simulink library "Custom_Valves"  (R2026a)
settings: Solver=VariableStepAuto
libraries: fl_lib x46, nesl_utility x7, MyMath_lib x2, SimscapeFluids_lib x2
Description:
  | Copyright 2020-2026 The MathWorks, Inc.
settings Model: Creator=smiller  LastModifiedBy=smiller

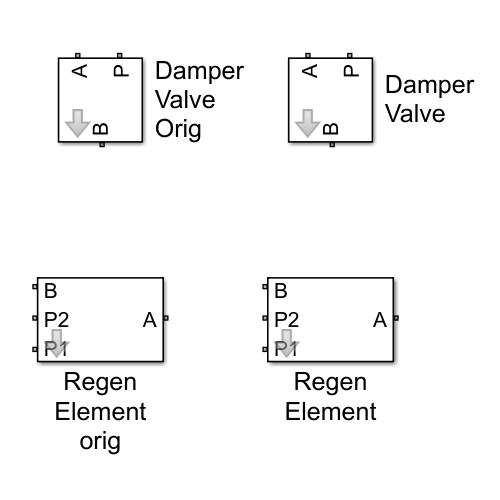
[thumbnail: Simulink's stored preview of the top-level diagram]
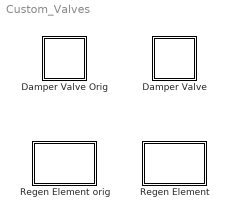
== system Custom_Valves ==
  Damper Valve : Subsystem  mask{sMax=valves.control.l.max, T=2e-2, AMax=orifices.sky.d1.s, pCrack=25, pMax=75}
      mask prompts: sMax "Maximum Valve Opening, in"; T "First-Order Time Lag, s"; AMax "Maximum Passage Area, in^2"; pCrack "Cracking Pressure, PSI"; pMax "Maximum Pressure, PSI"
      mask init:
      | % Calculate spring rate, k, assuming that the valve spring is the only
      | % element used to control the valve opening:
      | k = (pMax - pCrack)/sMax;
  Damper Valve Orig : Subsystem  mask{sMax=valves.control.l.max, T=2e-2, AMax=orifices.sky.d1.s, pCrack=25, pMax=75}
      mask prompts: sMax "Maximum Valve Opening, in"; T "First-Order Time Lag, s"; AMax "Maximum Passage Area, in^2"; pCrack "Cracking Pressure, PSI"; pMax "Maximum Pressure, PSI"
      mask init:
      | % Calculate spring rate, k, assuming that the valve spring is the only
      | % element used to control the valve opening:
      | k = (pMax - pCrack)/sMax;
  Regen Element : Subsystem  mask{sMax=valves.control.l.max, T=0.1, pCrack=1450, pMax=1550, AMax=lines.sky.c3.s.a, kA=1, kP1=3, kP2=1}
      mask prompts: sMax "Maximum Valve Opening, in"; T "First-Order Time Lag, s"; pCrack "Cracking Pressure, PSI"; pMax "Maximum Pressure, PSI"; AMax "Maximum Opening Area, in^2"; kA "Inlet Pilot Ratio"; kP1 "Rod End Pilot Ratio"; kP2 "Blind End Pilot Ratio"
      mask init:
      | % Calculate spring rate, k, assuming that the valve spring is the only
      | % element used to control the valve opening:
      | kS = (pMax - pCrack)/sMax;
  Regen Element orig : Subsystem  mask{sMax=valves.control.l.max, T=0.1, pCrack=1450, pMax=1550, AMax=lines.sky.c3.s.a, kA=1, kP1=3, kP2=1}
      mask prompts: sMax "Maximum Valve Opening, in"; T "First-Order Time Lag, s"; pCrack "Cracking Pressure, PSI"; pMax "Maximum Pressure, PSI"; AMax "Maximum Opening Area, in^2"; kA "Inlet Pilot Ratio"; kP1 "Rod End Pilot Ratio"; kP2 "Blind End Pilot Ratio"
      mask init:
      | % Calculate spring rate, k, assuming that the valve spring is the only
      | % element used to control the valve opening:
      | kS = (pMax - pCrack)/sMax;

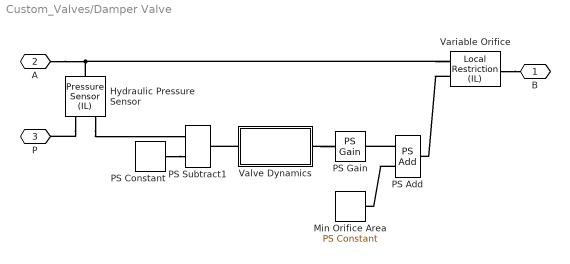
== system Custom_Valves/Damper Valve ==
  Hydraulic Pressure Sensor : fl_lib/Isothermal Liquid/Sensors/Pressure Sensor (IL)  pressure_measure=foundation.enum.pressure_measure.difference
  Min Orifice Area : fl_lib/Physical Signals/Sources/PS Constant  constant=2e-9 in^2
      settings: AttributesFormatString=%<constant> %<constant_unit>
  PS Add : fl_lib/Physical Signals/Functions/PS Add
  PS Constant : fl_lib/Physical Signals/Sources/PS Constant  constant=pCrack*6895 Pa
      settings: AttributesFormatString=%<constant> %<constant_unit>
  PS Gain : fl_lib/Physical Signals/Functions/PS Gain  gain=AMax/sMax in
  PS Subtract1 : fl_lib/Physical Signals/Functions/PS Subtract
  Valve Dynamics : Subsystem
  Variable Orifice : fl_lib/Isothermal Liquid/Elements/Local Restriction (IL)  restriction_type=foundation.enum.restriction_type.variable  restriction_area=1e-3 m^2  min_area=1e-9 in^2  max_area=1e10 m^2  area=inf m^2  Cd=0.7  Re_c=150  pressure_recovery=simscape.enum.onoff.off
  B : PMIOPort  Side=Right
  A : PMIOPort  Port=2  Side=Left
  P : PMIOPort  Port=3  Side=Left
  connections:
  A/RConn1 -- Variable Orifice/LConn1 -- Hydraulic Pressure Sensor/LConn1
  PS Constant/RConn1 -- PS Subtract1/LConn2
  Hydraulic Pressure Sensor/RConn2 -- PS Subtract1/LConn1
  Hydraulic Pressure Sensor/RConn1 -- P/RConn1
  PS Add/LConn2 -- Min Orifice Area/RConn1
  PS Gain/LConn1 -- Valve Dynamics/RConn1
  Valve Dynamics/LConn1 -- PS Subtract1/RConn1
  PS Add/LConn1 -- PS Gain/RConn1
  Variable Orifice/RConn1 -- B/RConn1
  Variable Orifice/LConn2 -- PS Add/RConn1

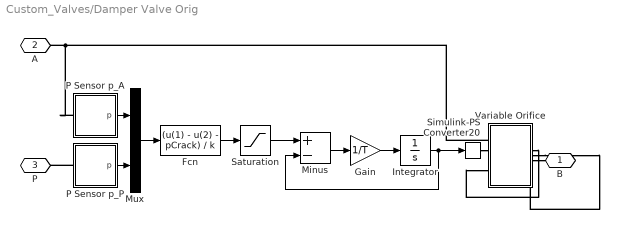
== system Custom_Valves/Damper Valve Orig ==
  Fcn : Fcn  Expr=(u(1) - u(2) - pCrack) / k
  Gain : Gain  Gain=1/T
  Integrator : Integrator
  Minus : Sum  Inputs=+-
  Mux : Mux  Inputs=2
  P Sensor p_A : Subsystem
  P Sensor p_P : Subsystem
  Saturation : Saturate  UpperLimit=sMax  LowerLimit=0
  Simulink-PS Converter20 : nesl_utility/Simulink-PS Converter  PhysicalDomain=network_engine_domain  SubClassName=ps_input  LeftPortType=input  RightPortType=output  PseudoPeriodic=off  Frequencies=[]  NoiseDistribution=none  NoiseParameters=[]  Unit=in  AffineConversion=off  FilteringAndDerivatives=provide  SimscapeFilterOrder=1  InputFilterTimeConstant=0.001  UdotUserProvided=0
  Variable Orifice : Subsystem
  B : PMIOPort  Side=Right
  A : PMIOPort  Port=2  Side=Left
  P : PMIOPort  Port=3  Side=Left
  wires:
  Integrator/1 -> Simulink-PS Converter20/1, Minus/2
  Gain/1 -> Integrator/1
  Minus/1 -> Gain/1
  Saturation/1 -> Minus/1
  Mux/1 -> Fcn/1
  P Sensor p_A/1(p) -> Mux/1
  P Sensor p_P/1(p) -> Mux/2
  Fcn/1 -> Saturation/1
  connections:
  P Sensor p_P/LConn1 -- P/RConn1
  A/RConn1 -- Variable Orifice/LConn1 -- P Sensor p_A/LConn1
  Simulink-PS Converter20/RConn1 -- Variable Orifice/LConn2
  Variable Orifice/RConn1 -- B/RConn1

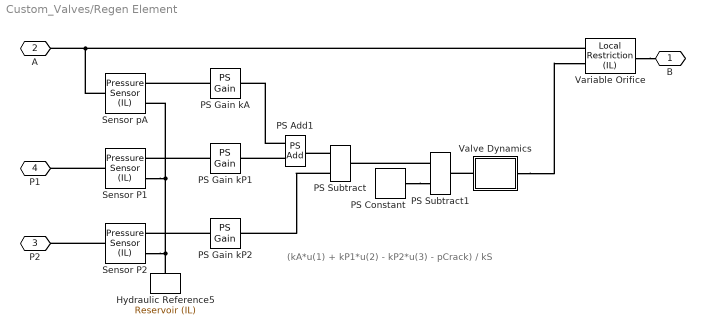
== system Custom_Valves/Regen Element ==
  note: (kA*u(1) + kP1*u(2) - kP2*u(3) - pCrack) / kS
  Hydraulic Reference5 : fl_lib/Isothermal Liquid/Elements/Reservoir (IL)  pressure_input=false  pressure_spec=foundation.enum.pressure_spec.atmospheric  reservoir_pressure=0.101325 MPa
  PS Add1 : fl_lib/Physical Signals/Functions/PS Add
  PS Constant : fl_lib/Physical Signals/Sources/PS Constant  constant=pCrack*6895 Pa
      settings: AttributesFormatString=%<constant> %<constant_unit>
  PS Gain kA : fl_lib/Physical Signals/Functions/PS Gain  gain=kA
      settings: AttributesFormatString=%<gain>
  PS Gain kP1 : fl_lib/Physical Signals/Functions/PS Gain  gain=kP1
      settings: AttributesFormatString=%<gain>
  PS Gain kP2 : fl_lib/Physical Signals/Functions/PS Gain  gain=kP2
      settings: AttributesFormatString=%<gain>
  PS Subtract : fl_lib/Physical Signals/Functions/PS Subtract
  PS Subtract1 : fl_lib/Physical Signals/Functions/PS Subtract
  Sensor P1 : fl_lib/Isothermal Liquid/Sensors/Pressure Sensor (IL)  pressure_measure=foundation.enum.pressure_measure.difference
  Sensor P2 : fl_lib/Isothermal Liquid/Sensors/Pressure Sensor (IL)  pressure_measure=foundation.enum.pressure_measure.difference
  Sensor pA : fl_lib/Isothermal Liquid/Sensors/Pressure Sensor (IL)  pressure_measure=foundation.enum.pressure_measure.difference
  Valve Dynamics : Subsystem
  Variable Orifice : fl_lib/Isothermal Liquid/Elements/Local Restriction (IL)  restriction_type=foundation.enum.restriction_type.variable  restriction_area=1e-3 m^2  min_area=1e-9 in^2  max_area=1e10 m^2  area=inf m^2  Cd=0.7  Re_c=150  pressure_recovery=simscape.enum.onoff.off
  B : PMIOPort  Side=Right
  A : PMIOPort  Port=2  Side=Left
  P2 : PMIOPort  Port=3  Side=Right
  P1 : PMIOPort  Port=4  Side=Right
  connections:
  Sensor P1/LConn1 -- P1/RConn1
  Sensor P2/LConn1 -- P2/RConn1
  PS Subtract1/LConn1 -- PS Subtract/RConn1
  PS Constant/RConn1 -- PS Subtract1/LConn2
  Hydraulic Reference5/LConn1 -- Sensor P2/RConn1 -- Sensor P1/RConn1 -- Sensor pA/RConn1
  PS Gain kA/LConn1 -- Sensor pA/RConn2
  PS Gain kP1/LConn1 -- Sensor P1/RConn2
  PS Gain kP2/LConn1 -- Sensor P2/RConn2
  PS Add1/LConn1 -- PS Gain kA/RConn1
  PS Add1/LConn2 -- PS Gain kP1/RConn1
  PS Subtract/LConn1 -- PS Add1/RConn1
  PS Subtract/LConn2 -- PS Gain kP2/RConn1
  Valve Dynamics/LConn1 -- PS Subtract1/RConn1
  Sensor pA/LConn1 -- Variable Orifice/LConn1 -- A/RConn1
  Variable Orifice/RConn1 -- B/RConn1
  Valve Dynamics/RConn1 -- Variable Orifice/LConn2

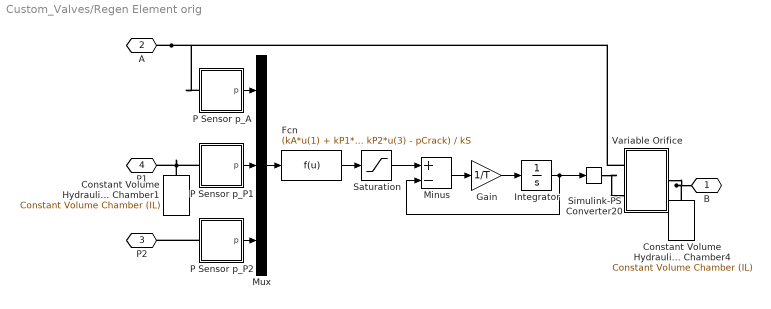
== system Custom_Valves/Regen Element orig ==
  Constant Volume Hydraulic Chamber1 : fl_lib/Isothermal Liquid/Elements/Constant Volume Chamber (IL)  volume=chamber.v in^3  p_I_specify=off  p_I_priority=High  p_I=0 + 101325 Pa  p_I_nominal_specify=off  p_I_nominal_value=1  p_I_nominal_unit=Pa
  Constant Volume Hydraulic Chamber4 : fl_lib/Isothermal Liquid/Elements/Constant Volume Chamber (IL)  volume=chamber.v in^3  p_I_specify=off  p_I_priority=High  p_I=0 + 101325 Pa  p_I_nominal_specify=off  p_I_nominal_value=1  p_I_nominal_unit=Pa
  Fcn : Fcn  Expr=(kA*u(1) + kP1*u(2) - kP2*u(3) - pCrack) / kS
  Gain : Gain  Gain=1/T
  Integrator : Integrator
  Minus : Sum  Inputs=+-
  Mux : Mux  Inputs=3
  P Sensor p_A : Subsystem
  P Sensor p_P1 : Subsystem
  P Sensor p_P2 : Subsystem
  Saturation : Saturate  UpperLimit=sMax  LowerLimit=0
  Simulink-PS Converter20 : nesl_utility/Simulink-PS Converter  PhysicalDomain=network_engine_domain  SubClassName=ps_input  LeftPortType=input  RightPortType=output  PseudoPeriodic=off  Frequencies=[]  NoiseDistribution=none  NoiseParameters=[]  Unit=in  AffineConversion=off  FilteringAndDerivatives=provide  SimscapeFilterOrder=1  InputFilterTimeConstant=0.001  UdotUserProvided=0
  Variable Orifice : Subsystem
  B : PMIOPort  Side=Right
  A : PMIOPort  Port=2  Side=Left
  P2 : PMIOPort  Port=3  Side=Right
  P1 : PMIOPort  Port=4  Side=Right
  wires:
  P Sensor p_P2/1(p) -> Mux/3
  Integrator/1 -> Simulink-PS Converter20/1, Minus/2
  Gain/1 -> Integrator/1
  Minus/1 -> Gain/1
  Saturation/1 -> Minus/1
  Mux/1 -> Fcn/1
  P Sensor p_A/1(p) -> Mux/1
  P Sensor p_P1/1(p) -> Mux/2
  Fcn/1 -> Saturation/1
  connections:
  P Sensor p_P2/LConn1 -- P2/RConn1
  Constant Volume Hydraulic Chamber1/LConn1 -- P1/RConn1 -- P Sensor p_P1/LConn1
  A/RConn1 -- Variable Orifice/LConn1 -- P Sensor p_A/LConn1
  B/RConn1 -- Variable Orifice/RConn1 -- Constant Volume Hydraulic Chamber4/LConn1
  Simulink-PS Converter20/RConn1 -- Variable Orifice/LConn2

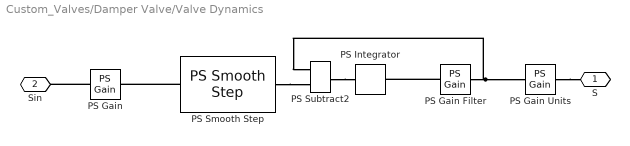
== system Custom_Valves/Damper Valve/Valve Dynamics ==
  PS Gain : fl_lib/Physical Signals/Functions/PS Gain  gain=1/k*0.000145038 1/Pa
      settings: AttributesFormatString=%<gain> %<gain_unit>
  PS Gain Filter : fl_lib/Physical Signals/Functions/PS Gain  gain=1/T 1/s
      settings: AttributesFormatString=%<gain> %<gain_unit>
  PS Gain Units : fl_lib/Physical Signals/Functions/PS Gain  gain=1 in
  PS Integrator : fl_lib/Physical Signals/Linear Operators/PS Integrator  reset_method=foundation.enum.IntegratorResetSpec.None  initial_condition_spec=foundation.enum.IntegratorICSpec.Internal  saturation_spec=foundation.enum.IntegratorSaturationSpec.None  saturation_source_spec=foundation.enum.IntegratorSaturationSourceSpec.Internal  x0=0*T s  xu=inf s  xl=-inf s
      settings: AttributesFormatString=%<x0> %<x0_unit>
  PS Smooth Step : MyMath_lib/PS Smooth Step  step_start=0  step_finish=sMax  min_out=0  max_out=sMax
  PS Subtract2 : fl_lib/Physical Signals/Functions/PS Subtract
  S : PMIOPort  Side=Right
  Sin : PMIOPort  Port=2  Side=Left
  connections:
  PS Smooth Step/LConn1 -- PS Gain/RConn1
  PS Smooth Step/RConn1 -- PS Subtract2/LConn1
  PS Gain Units/RConn1 -- S/RConn1
  PS Gain Filter/RConn1 -- PS Subtract2/LConn2 -- PS Gain Units/LConn1
  PS Subtract2/RConn1 -- PS Integrator/LConn1
  PS Gain Filter/LConn1 -- PS Integrator/RConn1
  PS Gain/LConn1 -- Sin/RConn1

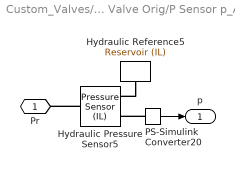
== system Custom_Valves/Damper Valve Orig/P Sensor p_A ==
  Hydraulic Pressure Sensor5 : fl_lib/Isothermal Liquid/Sensors/Pressure Sensor (IL)  pressure_measure=foundation.enum.pressure_measure.difference
  Hydraulic Reference5 : fl_lib/Isothermal Liquid/Elements/Reservoir (IL)  pressure_input=false  pressure_spec=foundation.enum.pressure_spec.atmospheric  reservoir_pressure=0.101325 MPa
  PS-Simulink Converter20 : nesl_utility/PS-Simulink Converter  PhysicalDomain=network_engine_domain  SubClassName=ps_output  LeftPortType=input  RightPortType=output  PseudoPeriodic=off  Frequencies=[]  VectorFormat=1-D array  Unit=psi  AffineConversion=off
  Pr : PMIOPort  Side=Left
  p : Outport
  wires:
  PS-Simulink Converter20/1 -> p/1
  connections:
  Hydraulic Pressure Sensor5/LConn1 -- Pr/RConn1
  Hydraulic Reference5/LConn1 -- Hydraulic Pressure Sensor5/RConn1
  PS-Simulink Converter20/LConn1 -- Hydraulic Pressure Sensor5/RConn2

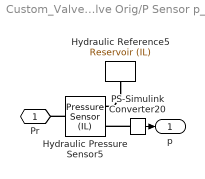
== system Custom_Valves/Damper Valve Orig/P Sensor p_P ==
  Hydraulic Pressure Sensor5 : fl_lib/Isothermal Liquid/Sensors/Pressure Sensor (IL)  pressure_measure=foundation.enum.pressure_measure.difference
  Hydraulic Reference5 : fl_lib/Isothermal Liquid/Elements/Reservoir (IL)  pressure_input=false  pressure_spec=foundation.enum.pressure_spec.atmospheric  reservoir_pressure=0.101325 MPa
  PS-Simulink Converter20 : nesl_utility/PS-Simulink Converter  PhysicalDomain=network_engine_domain  SubClassName=ps_output  LeftPortType=input  RightPortType=output  PseudoPeriodic=off  Frequencies=[]  VectorFormat=1-D array  Unit=psi  AffineConversion=off
  Pr : PMIOPort  Side=Left
  p : Outport
  wires:
  PS-Simulink Converter20/1 -> p/1
  connections:
  PS-Simulink Converter20/LConn1 -- Hydraulic Pressure Sensor5/RConn2
  Hydraulic Reference5/LConn1 -- Hydraulic Pressure Sensor5/RConn1
  Hydraulic Pressure Sensor5/LConn1 -- Pr/RConn1

== system Custom_Valves/Damper Valve Orig/Variable Orifice ==
  Variable Orifice : SimscapeFluids_lib/Isothermal Liquid/Valves & Orifices/Orifices/Orifice (IL)  orifice_type=foundation.enum.constant_variable.variable  constant_orifice_spec=fluids.isothermal_liquid.valves_orifices.orifices.enum.constant_orifice_spec.area  variable_orifice_spec=1  orifice_area_constant=1e-3 m^2  p_diff_TLU_constant=[-4, -3, -2, -1, -.5, 0, .5, 1, 2, 3, 4] MPa  vol_flow_TLU_constant=[-2.44, -2.12, -1.68, -1.22, -.84, 0, .85, 1.21, 1.7, 2.09, 2.41] .* 1e-3 m^3/s  S_min=(sMax)/(AMax)*(1e-12) - 0.0254*(0) m^2/in  del_S=0.00064516*(-39.3701*(0) + (sMax)) - ((sMax)/(AMax)*(1e-12) - 0.0254*(0)) m^2/in  open_orientation=1  area_max=AMax in^2  area_leak=1e-12 m^2  S_TLU=[-.002, 0, .002, .005, .015] - (0) m  orifice_area_TLU=[1e-09, 2.0352e-07, 4.0736e-05, .00011438, .00034356] m^2  area=inf m^2  Cd=0.7  Re_c=150  smoothing_factor=0  pressure_recovery=false  S_vol_flow_TLU=[-.002, 0, .002, .005, .015] - (0) m  p_diff_TLU=[-10000000, -5000000, -2000000, 2000000, 5000000, 10000000] Pa  vol_flow_TLU=[-1e-07, -7.0711e-08, -4.4721e-08, 4.4721e-08, 7.0711e-08, 1e-07; -2.0352e-05, -1.4391e-05, -9.1017e-06, 9.1017e-06, 1.4391e-05, 2.0352e-05; -.0040736, -.0028805, -.0018218, .0018218, .0028805, .0040736; -.011438, -.0080879, -.0051152, .0051152, .0080879, .011438; -.034356, -.024293, -.015364, .015364, .024293, .034356] m^3/s
  A : PMIOPort  Side=Left
  S : PMIOPort  Port=2  Side=Left
  B : PMIOPort  Port=3  Side=Right
  connections:
  S/RConn1 -- Variable Orifice/LConn2
  A/RConn1 -- Variable Orifice/LConn1
  Variable Orifice/RConn1 -- B/RConn1

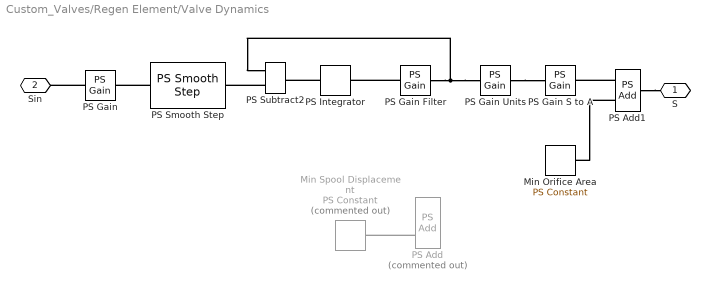
== system Custom_Valves/Regen Element/Valve Dynamics ==
  Min Orifice Area : fl_lib/Physical Signals/Sources/PS Constant  constant=2e-7 in^2
      settings: AttributesFormatString=%<constant> %<constant_unit>
  Min Spool Displacement : fl_lib/Physical Signals/Sources/PS Constant  Commented=on  constant=1e-6 in
      settings: AttributesFormatString=%<constant> %<constant_unit>
  PS Add : fl_lib/Physical Signals/Functions/PS Add  Commented=on
  PS Add1 : fl_lib/Physical Signals/Functions/PS Add
  PS Gain : fl_lib/Physical Signals/Functions/PS Gain  gain=1/kS*0.000145038 1/Pa
      settings: AttributesFormatString=%<gain>
  PS Gain S to A : fl_lib/Physical Signals/Functions/PS Gain  gain=AMax/sMax in
  PS Gain Filter : fl_lib/Physical Signals/Functions/PS Gain  gain=1/T 1/s
      settings: AttributesFormatString=%<gain> %<gain_unit>
  PS Gain Units : fl_lib/Physical Signals/Functions/PS Gain  gain=1 in
  PS Integrator : fl_lib/Physical Signals/Linear Operators/PS Integrator  reset_method=foundation.enum.IntegratorResetSpec.None  initial_condition_spec=foundation.enum.IntegratorICSpec.Internal  saturation_spec=foundation.enum.IntegratorSaturationSpec.None  saturation_source_spec=foundation.enum.IntegratorSaturationSourceSpec.Internal  x0=0*T s  xu=inf s  xl=-inf s
      settings: AttributesFormatString=IC: %<x0> %<x0_unit>
  PS Smooth Step : MyMath_lib/PS Smooth Step  step_start=0  step_finish=sMax  min_out=0  max_out=sMax
  PS Subtract2 : fl_lib/Physical Signals/Functions/PS Subtract
  S : PMIOPort  Side=Right
  Sin : PMIOPort  Port=2  Side=Left
  connections:
  PS Gain Filter/LConn1 -- PS Integrator/RConn1
  PS Integrator/LConn1 -- PS Subtract2/RConn1
  PS Add/LConn2 -- Min Spool Displacement/RConn1
  PS Subtract2/LConn1 -- PS Smooth Step/RConn1
  PS Smooth Step/LConn1 -- PS Gain/RConn1
  PS Gain/LConn1 -- Sin/RConn1
  PS Gain Units/RConn1 -- PS Gain S to A/LConn1
  PS Add1/RConn1 -- S/RConn1
  PS Gain Units/LConn1 -- PS Gain Filter/RConn1 -- PS Subtract2/LConn2
  PS Add1/LConn1 -- PS Gain S to A/RConn1
  PS Add1/LConn2 -- Min Orifice Area/RConn1

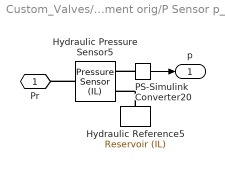
== system Custom_Valves/Regen Element orig/P Sensor p_A ==
  Hydraulic Pressure Sensor5 : fl_lib/Isothermal Liquid/Sensors/Pressure Sensor (IL)  pressure_measure=foundation.enum.pressure_measure.difference
  Hydraulic Reference5 : fl_lib/Isothermal Liquid/Elements/Reservoir (IL)  pressure_input=false  pressure_spec=foundation.enum.pressure_spec.atmospheric  reservoir_pressure=0.101325 MPa
  PS-Simulink Converter20 : nesl_utility/PS-Simulink Converter  PhysicalDomain=network_engine_domain  SubClassName=ps_output  LeftPortType=input  RightPortType=output  PseudoPeriodic=off  Frequencies=[]  VectorFormat=1-D array  Unit=psi  AffineConversion=off
  Pr : PMIOPort  Side=Left
  p : Outport
  wires:
  PS-Simulink Converter20/1 -> p/1
  connections:
  Hydraulic Pressure Sensor5/LConn1 -- Pr/RConn1
  Hydraulic Reference5/LConn1 -- Hydraulic Pressure Sensor5/RConn1
  PS-Simulink Converter20/LConn1 -- Hydraulic Pressure Sensor5/RConn2

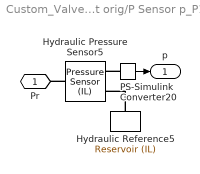
== system Custom_Valves/Regen Element orig/P Sensor p_P1 ==
  Hydraulic Pressure Sensor5 : fl_lib/Isothermal Liquid/Sensors/Pressure Sensor (IL)  pressure_measure=foundation.enum.pressure_measure.difference
  Hydraulic Reference5 : fl_lib/Isothermal Liquid/Elements/Reservoir (IL)  pressure_input=false  pressure_spec=foundation.enum.pressure_spec.atmospheric  reservoir_pressure=0.101325 MPa
  PS-Simulink Converter20 : nesl_utility/PS-Simulink Converter  PhysicalDomain=network_engine_domain  SubClassName=ps_output  LeftPortType=input  RightPortType=output  PseudoPeriodic=off  Frequencies=[]  VectorFormat=1-D array  Unit=psi  AffineConversion=off
  Pr : PMIOPort  Side=Left
  p : Outport
  wires:
  PS-Simulink Converter20/1 -> p/1
  connections:
  Hydraulic Pressure Sensor5/LConn1 -- Pr/RConn1
  Hydraulic Reference5/LConn1 -- Hydraulic Pressure Sensor5/RConn1
  PS-Simulink Converter20/LConn1 -- Hydraulic Pressure Sensor5/RConn2

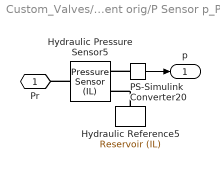
== system Custom_Valves/Regen Element orig/P Sensor p_P2 ==
  Hydraulic Pressure Sensor5 : fl_lib/Isothermal Liquid/Sensors/Pressure Sensor (IL)  pressure_measure=foundation.enum.pressure_measure.difference
  Hydraulic Reference5 : fl_lib/Isothermal Liquid/Elements/Reservoir (IL)  pressure_input=false  pressure_spec=foundation.enum.pressure_spec.atmospheric  reservoir_pressure=0.101325 MPa
  PS-Simulink Converter20 : nesl_utility/PS-Simulink Converter  PhysicalDomain=network_engine_domain  SubClassName=ps_output  LeftPortType=input  RightPortType=output  PseudoPeriodic=off  Frequencies=[]  VectorFormat=1-D array  Unit=psi  AffineConversion=off
  Pr : PMIOPort  Side=Left
  p : Outport
  wires:
  PS-Simulink Converter20/1 -> p/1
  connections:
  PS-Simulink Converter20/LConn1 -- Hydraulic Pressure Sensor5/RConn2
  Hydraulic Reference5/LConn1 -- Hydraulic Pressure Sensor5/RConn1
  Hydraulic Pressure Sensor5/LConn1 -- Pr/RConn1

== system Custom_Valves/Regen Element orig/Variable Orifice ==
  Variable Orifice : SimscapeFluids_lib/Isothermal Liquid/Valves & Orifices/Orifices/Orifice (IL)  orifice_type=foundation.enum.constant_variable.variable  constant_orifice_spec=fluids.isothermal_liquid.valves_orifices.orifices.enum.constant_orifice_spec.area  variable_orifice_spec=1  orifice_area_constant=1e-3 m^2  p_diff_TLU_constant=[-4, -3, -2, -1, -.5, 0, .5, 1, 2, 3, 4] MPa  vol_flow_TLU_constant=[-2.44, -2.12, -1.68, -1.22, -.84, 0, .85, 1.21, 1.7, 2.09, 2.41] .* 1e-3 m^3/s  S_min=(sMax)/(AMax)*(1e-12) - 0.0254*(0) m^2/in  del_S=0.00064516*(-39.3701*(0) + (sMax)) - ((sMax)/(AMax)*(1e-12) - 0.0254*(0)) m^2/in  open_orientation=1  area_max=AMax in^2  area_leak=1e-12 m^2  S_TLU=[-.002, 0, .002, .005, .015] - (0) m  orifice_area_TLU=[1e-09, 2.0352e-07, 4.0736e-05, .00011438, .00034356] m^2  area=inf m^2  Cd=0.7  Re_c=150  smoothing_factor=0  pressure_recovery=false  S_vol_flow_TLU=[-.002, 0, .002, .005, .015] - (0) m  p_diff_TLU=[-10000000, -5000000, -2000000, 2000000, 5000000, 10000000] Pa  vol_flow_TLU=[-1e-07, -7.0711e-08, -4.4721e-08, 4.4721e-08, 7.0711e-08, 1e-07; -2.0352e-05, -1.4391e-05, -9.1017e-06, 9.1017e-06, 1.4391e-05, 2.0352e-05; -.0040736, -.0028805, -.0018218, .0018218, .0028805, .0040736; -.011438, -.0080879, -.0051152, .0051152, .0080879, .011438; -.034356, -.024293, -.015364, .015364, .024293, .034356] m^3/s
  A : PMIOPort  Side=Left
  S : PMIOPort  Port=2  Side=Left
  B : PMIOPort  Port=3  Side=Right
  connections:
  A/RConn1 -- Variable Orifice/LConn1
  Variable Orifice/RConn1 -- B/RConn1
  S/RConn1 -- Variable Orifice/LConn2
